simulink model "week1_problem8"  (R2020b)
settings: Solver=VariableStepAuto  StartTime=0.0  StopTime=10.0  RelTol=1e-3
settings Model: Creator=gokul  LastModifiedBy=gokul

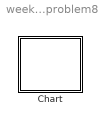
== system week1_problem8 ==
  Chart : Stateflow chart  TreatAsAtomicUnit=on

== stateflow chart week1_problem8/Chart ==
  state LiftFunctionOn
    state GroundFloor
      entry:
      status=1;
      during:
      CurrentFloor=0;
      FloorCheck(CurrentFloor);
      exit:
      status=0;
    state FirstFloor
      entry:
      status=1;
      during:
      CurrentFloor=1;
      FloorCheck(CurrentFloor);
      exit:
      status=0;
    state SecondFloor
      entry:
      status=1;
      during:
      CurrentFloor=2;
      FloorCheck(CurrentFloor);
      exit:
      status=0;
      after(1,sec);
    state ThirdFloor
      entry:
      status=1;
      during:
      CurrentFloor=3;
      FloorCheck(CurrentFloor);
      exit:
      status=0;
      after(1,sec);
    state FourthFloor
      entry:
      status=1;
      during:
      CurrentFloor=4;
      FloorCheck(CurrentFloor);
      exit:
      status=0;
    state FifthFloor
      entry:
      status=1;
      during:
      CurrentFloor=5;
      FloorCheck(CurrentFloor);
      exit:
      status=0;
    (default) -> GroundFloor
    GroundFloor -> FirstFloor
    FirstFloor -> GroundFloor [order 2]
    FirstFloor -> SecondFloor [order 1]
    SecondFloor -> FirstFloor [order 2]
    SecondFloor -> ThirdFloor [order 1]
    ThirdFloor -> SecondFloor [order 2]
    ThirdFloor -> FourthFloor [order 1]
    FourthFloor -> ThirdFloor [order 2]
    FourthFloor -> FifthFloor [order 1]
    FifthFloor -> FourthFloor
  (default) -> LiftFunctionOn
